simulink model "mohu_demo1"  (R2018b)
settings: Solver=VariableStepAuto  StartTime=0.0  StopTime=15  RelTol=1e-3
model workspace (MAT data in the model file):
  TC = 0.05
libraries: Solver_SF x1, simulink x1
settings Model: Creator=Hiro  LastModifiedBy=Hiro

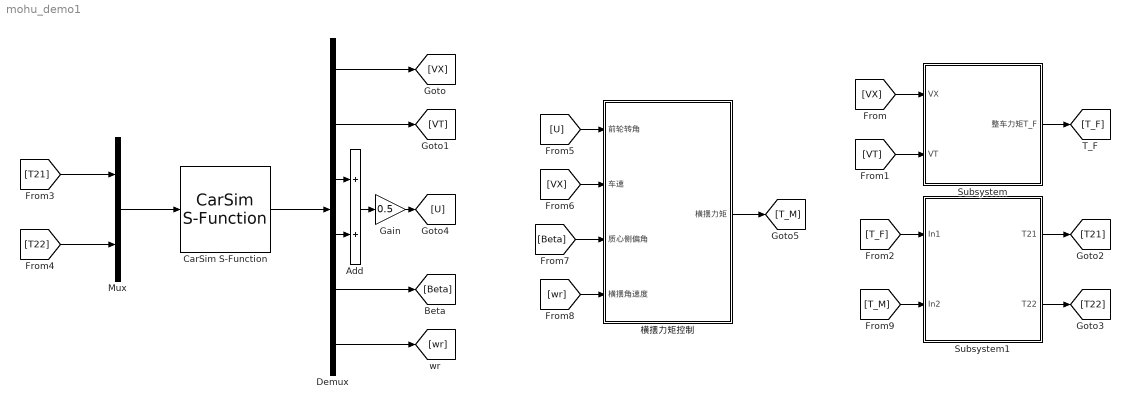
== system mohu_demo1 ==
  Add : Sum
  CarSim S-Function : Solver_SF/CarSim S-Function  Priority=1  SIMFILE=simfile.sim  Run_RTs=off  vs_state_ind=Run  StopMode_ind=Vehicle Model
  Demux : Demux  Outputs=6
  Gain : Gain  Gain=0.5
  Mux : Mux  Inputs=2
  Subsystem : Subsystem
  Subsystem1 : Subsystem
  横摆力矩控制 : Subsystem
  wires:
  Mux/1 -> CarSim S-Function/1
  CarSim S-Function/1 -> Demux/1
  Demux/1 -> [VX]
  Demux/2 -> [VT]
  [VX] -> Subsystem/1(VX)
  [VT] -> Subsystem/2(VT)
  Subsystem/1(整车力矩T_F) -> [T_F]
  [T_F] -> Subsystem1/1(In1)
  Subsystem1/1(T21) -> [T21]
  Subsystem1/2(T22) -> [T22]
  [T21] -> Mux/1
  [T22] -> Mux/2
  Demux/4 -> Add/2
  Demux/3 -> Add/1
  Add/1 -> Gain/1
  Gain/1 -> [U]
  Demux/6 -> [wr]
  Demux/5 -> [Beta]
  [U] -> 横摆力矩控制/1(前轮转角)
  [VX] -> 横摆力矩控制/2(车速)
  [Beta] -> 横摆力矩控制/3(质心侧偏角)
  [wr] -> 横摆力矩控制/4(横摆角速度)
  横摆力矩控制/1(横摆力矩) -> [T_M]
  [T_M] -> Subsystem1/2(In2)

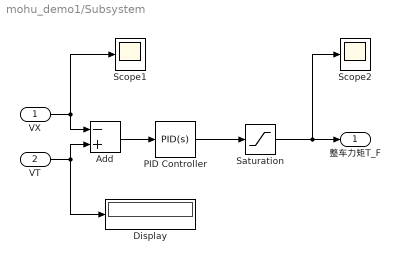
== system mohu_demo1/Subsystem ==
  VX : Inport
  VT : Inport  Port=2
  Add : Sum  Inputs=-+
  Display : Display
  PID Controller : simulink/Continuous/PID Controller  Controller=PID  Form=Parallel  TimeDomain=Continuous-time  SampleTime=-1  IntegratorMethod=Forward Euler  FilterMethod=Forward Euler  ControllerParametersSource=internal  P=300  I=300  D=10  UseFilter=on  N=100  TunerSelectOption=Transfer Function Based (PID Tuner App)  InitialConditionSource=internal  InitialConditionForIntegrator=0  InitialConditionForFilter=0  DifferentiatorICPrevScaledInput=0  ExternalReset=none  TrackingMode=off  Kt=1  LimitOutput=off  UpperSaturationLimit=inf  LowerSaturationLimit=-inf  LinearizeAsGain=on  AntiWindupMode=none  Kb=1  POutMin=[]  POutMax=[]  IOutMin=[]  IOutMax=[]  DOutMin=[]  DOutMax=[]  NOutMin=[]  NOutMax=[]  SumOutMin=[]  SumOutMax=[]  SaturationOutMin=[]  SaturationOutMax=[]  PParamMin=[]  PParamMax=[]  IParamMin=[]  IParamMax=[]  DParamMin=[]  DParamMax=[]  NParamMin=[]  NParamMax=[]  KbParamMin=[]  KbParamMax=[]  KtParamMin=[]  KtParamMax=[]  KbOutMin=[]  KbOutMax=[]  KtOutMin=[]  KtOutMax=[]  IntegratorOutMin=[]  IntegratorOutMax=[]  FilterOutMin=[]  FilterOutMax=[]  SumI1OutMin=[]  SumI1OutMax=[]  SumI2OutMin=[]  SumI2OutMax=[]  SumI3OutMin=[]  SumI3OutMax=[]  SumI4OutMin=[]  SumI4OutMax=[]  SumDOutMin=[]  SumDOutMax=[]  DifferentiatorOutMin=[]  DifferentiatorOutMax=[]  FilterDiffOutCoefMin=[]  FilterDiffOutCoefMax=[]  ReciprocalOutMin=[]  ReciprocalOutMax=[]  SumDenOutMin=[]  SumDenOutMax=[]  SumNumOutMin=[]  SumNumOutMax=[]  DivideOutMin=[]  DivideOutMax=[]  IntegratorContinuousStateAttributes=''  IntegratorStateMustResolveToSignalObject=off  IntegratorRTWStateStorageClass=Auto  FilterContinuousStateAttributes=''  FilterStateMustResolveToSignalObject=off  FilterRTWStateStorageClass=Auto  ParallelPVariant=InternalParameters  IdealPVariant=Disabled  IVariant=InternalParameters  DVariant=InternalParameters  IntegratorVariant=Continuous  SatVariant=Disabled  AWVariant=Passthrough  PCopyVariant=Disabled  TRVariant=Disabled  FdbkBlocksVariant=Forward  IdealPFdbkVariant=Disabled  SatFdbkVariant=Disabled  DerivativeFilterVariant=ContFilter  NVariant=InternalParameters  NCopyVariant=Disabled  FilterICVariant=InternalICsFilter  IntegratorICVariant=InternalICs  ExternalResetVariant=Disabled  TRSumVariant=Passthrough  SumFdbkVariant=Disabled  SumVariant=Sum_PID
  Saturation : Saturate  UpperLimit=280  LowerLimit=0
  Scope1 : Scope
  Scope2 : Scope
  整车力矩T_F : Outport
  wires:
  VX/1 -> Scope1/1, Add/1
  VT/1 -> Display/1, Add/2
  Add/1 -> PID Controller/1
  PID Controller/1 -> Saturation/1
  Saturation/1 -> Scope2/1, 整车力矩T_F/1

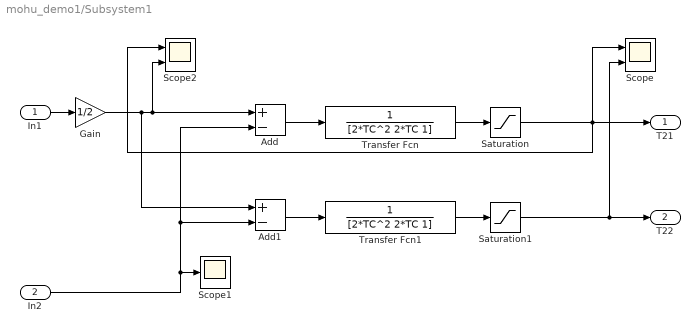
== system mohu_demo1/Subsystem1 ==
  In1 : Inport
  In2 : Inport  Port=2
  Add : Sum  Inputs=+-
  Add1 : Sum  Inputs=+-
  Gain : Gain  Gain=1/2
  Saturation : Saturate  UpperLimit=140  LowerLimit=0
  Saturation1 : Saturate  UpperLimit=140  LowerLimit=0
  Scope : Scope  NumInputPorts=2
  Scope1 : Scope
  Scope2 : Scope  NumInputPorts=2
  Transfer Fcn : TransferFcn  Denominator=[2*TC^2 2*TC 1]
  Transfer Fcn1 : TransferFcn  Denominator=[2*TC^2 2*TC 1]
  T21 : Outport
  T22 : Outport  Port=2
  wires:
  In1/1 -> Gain/1
  Transfer Fcn/1 -> Saturation/1
  Transfer Fcn1/1 -> Saturation1/1
  Gain/1 -> Add/1, Scope2/2, Add1/1
  In2/1 -> Add/2, Add1/2, Scope1/1
  Add1/1 -> Transfer Fcn1/1
  Add/1 -> Transfer Fcn/1
  Saturation/1 -> Scope2/1, Scope/1, T21/1
  Saturation1/1 -> Scope/2, T22/1

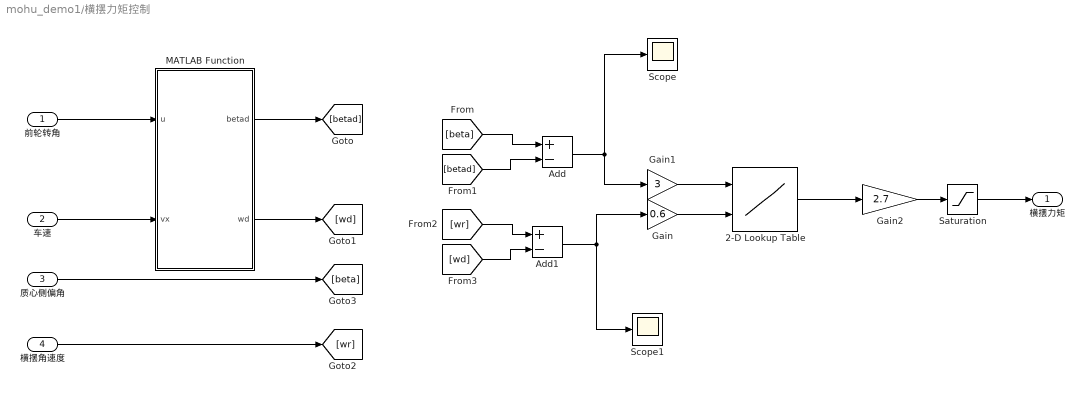
== system mohu_demo1/横摆力矩控制 ==
  前轮转角 : Inport
  车速 : Inport  Port=2
  质心侧偏角 : Inport  Port=3
  横摆角速度 : Inport  Port=4
  2-D Lookup Table : Lookup_n-D  BreakpointsForDimension1=[1:10]  BreakpointsForDimension2=[1:21]  Table="[0\t0\t0\t0\t0\t0\t0\t0\t0\t0\t0\t0\t0\t0\t0\t0\t0\t0\t0\t0\t0;0\t1.40000000000000\t1.40000000000000\t1.40000000000000\t1.80000000000000\t2.70000000000000\t3.60000000000000\t3.60000000000000\t3.60000000000000\t3.60000000000000\t3.60000000000000\t3.60000000000000\t4.10000000000000\t4.80000000000000\t5.40000000000000\t5.40000000000000\t5.40000000000000\t5.40000000000000\t5.40000000000000\t5.40000000000000\t5.40000000000000;0\t1.50000000000000\t1.50000000000000\t1.50000000000000\t2.10000000000000\t2.60000000000000\t3.60000000000000\t3.60000000000000\t3.60000000000000\t4.10000000000000\t4.60000000000000\t5.40000000000000\t5.40000000000000\t5.40000000000000\t5.40000000000000\t5.40000000000000\t5.40000000000000\t5.40000000000000\t5.40000000000000\t5.40000000000000\t5.40000000000000;0\t1.50000000000000\t1.50000000000000\t1.50000000000000\t2.10000000000000\t2.60000000000000\t3.60000000000000\t3.60000000000000\t3.60000000000000\t4.10000000000000\t4.60000000000000\t5.40000000000000\t5.40000000000000\t5.40000000000000\t5.40000000000000\t5.40000000000000\t5.40000000000000\t5.40000000000000\t5.40000000000000\t5.40000000000000\t5.40000000000000;0\t1.40000000000000\t1.40000000000000\t1.40000000000000\t1.80000000000000\t2.70000000000000\t3.60000000000000\t4.40000000000000\t5\t5.40000000000000\t5.40000000000000\t5.40000000000000\t5.90000000000000\t6.60000000000000\t7.20000000000000\t7.20000000000000\t7.20000000000000\t7.20000000000000\t7.20000000000000\t7.20000000000000\t7.20000000000000;0\t1.50000000000000\t1.50000000000000\t1.50000000000000\t2.10000000000000\t2.60000000000000\t3.60000000000000\t4.40000000000000\t4.90000000000000\t5.90000000000000\t6.40000000000000\t7.20000000000000\t9.20000000000000\t10.5000000000000\t11.1000000000000\t11.1000000000000\t11.1000000000000\t11.1000000000000\t11.1000000000000\t11.1000000000000\t11.1000000000000;0\t1.50000000000000\t1.50000000000000\t1.50000000000000\t2.10000000000000\t2.60000000000000\t3.60000000000000\t4.40000000000000\t4.90000000000000\t5.90000000000000\t6.40000000000000\t7.20000000000000\t9.20000000000000\t10.5000000000000\t11.1000000000000\t11.1000000000000\t11.1000000000000\t11.1000000000000\t11.1000000000000\t11.1000000000000\t11.1000000000000;0\t1.50000000000000\t1.50000000000000\t1.50000000000000\t2.70000000000000\t3.50000000000000\t5.40000000000000\t6.20000000000000\t6.70000000000000\t9.20000000000000\t10.3000000000000\t11.1000000000000\t11.1000000000000\t11\t11.1000000000000\t11.1000000000000\t11.1000000000000\t11.1000000000000\t11.1000000000000\t11.1000000000000\t11.1000000000000;0\t1.40000000000000\t1.40000000000000\t1.40000000000000\t2.30000000000000\t3.60000000000000\t5.40000000000000\t6.20000000000000\t6.80000000000000\t9\t10.4000000000000\t11.3000000000000\t11.1000000000000\t11\t11.1000000000000\t11.2000000000000\t11.3000000000000\t11.3000000000000\t11.3000000000000\t11.3000000000000\t11.3000000000000;0\t1.40000000000000\t1.40000000000000\t1.40000000000000\t2.30000000000000\t3.60000000000000\t5.40000000000000\t6.20000000000000\t6.80000000000000\t9\t10.4000000000000\t11.3000000000000\t11.1000000000000\t11\t11.1000000000000\t11.2000000000000\t11.3000000000000\t11.3000000000000\t11.3000000000000\t11.3000000000000\t11.3000000000000]"  InternalRulePriority=Speed  RndMeth=Simplest  InputSameDT=on
  Add : Sum  Inputs=+-
  Add1 : Sum  Inputs=+-
  Gain : Gain  Gain=0.6
  Gain1 : Gain  Gain=3
  Gain2 : Gain  Gain=2.7
  MATLAB Function : MATLAB Function  TreatAsAtomicUnit=on
  Saturation : Saturate  UpperLimit=140  LowerLimit=0
  Scope : Scope
  Scope1 : Scope
  横摆力矩 : Outport
  wires:
  车速/1 -> MATLAB Function/2(vx)
  前轮转角/1 -> MATLAB Function/1(u)
  MATLAB Function/2(wd) -> [wd]
  MATLAB Function/1(betad) -> [betad]
  横摆角速度/1 -> [wr]
  质心侧偏角/1 -> [beta]
  [beta] -> Add/1
  [betad] -> Add/2
  [wr] -> Add1/1
  [wd] -> Add1/2
  Add1/1 -> Gain/1, Scope1/1
  Add/1 -> Gain1/1, Scope/1
  2-D Lookup Table/1 -> Gain2/1
  Gain/1 -> 2-D Lookup Table/2
  Gain1/1 -> 2-D Lookup Table/1
  Gain2/1 -> Saturation/1
  Saturation/1 -> 横摆力矩/1

== matlab function mohu_demo1/横摆力矩控制/MATLAB Function ==
  data: u input; betad output; vx input; wd output
function [betad,wd] = fcn(u,vx)
%%
m=275+70;%整车质量
a=1.015;%质心到前轴距离
b=1.895;%质心到后轴的距离
Bf=1.539;%前轮轴距
Br=1.539;%后轮轴距
r=0.325;%轮胎有效滚动半径
L=a+b;%轴距
miu=0.85;%路面附着系数
g=9.81;%重力加速度
Iz=1536.7;%绕z轴转动惯量
k1=-112600;%前轴侧偏刚度
k2=-89500;%后轴侧偏刚度
vx=120/3.6;
A1=[(k1+k2)/m/vx (a*k1-b*k2)/m/vx/vx-1;(a*k1-b*k2)/Iz (a*a*k1+b*b*k2)/Iz/vx];%2DOF状态空间方程A矩阵
B1=[-k1/m/vx;-a*k1/Iz];%2DOF状态空间方程B矩阵
C=[(k1+k2)/m (a*k1-b*k2)/m/vx;0 1];
D=[-k1/m;0];
Q=diag([0.01,0.01]);
k=m*(a/k2-b/k1)/L/L;%稳定性因素
wd1=vx/L/(1+k*vx^2)*u;
betad=0;
if  abs(wd1)<=abs(0.85*miu*g/vx)
    wd=wd1;
else
    wd=0.85*miu*g/vx*sign(u);
end
